simulink model "inanout"  (R2018a)
settings: Solver=FixedStepDiscrete  StartTime=0.0  StopTime=10.0  FixedStep=1e-4  RelTol=1e-3
InitFcn:
  | mbd_pnt_consistency_checks(bdroot(gcs));
undefined symbols (not defined in the file): B14, C10
libraries: mbd_pnt_ec_toolbox x6, simulink x2
settings Model: Creator=oolonthegreat  LastModifiedBy=oolonthegreat
settings DataIOCC: ExternalInput=off  InitialState=off  SaveOutput=off  SignalLogging=off  SaveTime=off
settings OptimizationCC: DefaultParameterBehavior=Inlined  EnhancedBackFolding=on  PassReuseOutputArgsAs=Individual arguments  OptimizeBlockOrder=speed  DifferentSizesBufferReuse=on  OptimizationCustomize=off
settings DebuggingCC: InheritedTsInSrcMsg=none  SingleTaskRateTransMsg=error  ParameterTunabilityLossMsg=error  UnconnectedInputMsg=error  UnconnectedOutputMsg=error  UnconnectedLineMsg=error  UnknownTsInhSupMsg=error
settings HardwareCC: ProdBitPerPointer=32  ProdBitPerSizeT=32  ProdBitPerPtrDiffT=32  ProdLargestAtomicInteger=Long  ProdLargestAtomicFloat=Double  ProdEndianess=BigEndian  ProdWordSize=32  ProdHWDeviceType=Motorola PowerPC
settings SFSimCC: MATLABDynamicMemAlloc=off
settings RTWCC: SystemTargetFile=mbd_pnt.tlc  MakeCommand=mbd_pnt_make_rtw COPY_MDLREF_INCLUDES=0  TemplateMakefile=mbd_pnt.tmf  PostCodeGenCommand=mbd_pnt_analyzegencode(buildInfo)  Description=Model Based Design Toolbox MPC574xP Code Generation Target  GenerateReport=on  IncludeHyperlinkInReport=on  LaunchReport=on  GenerateTraceInfo=on  GenerateTraceReport=on  GenerateTraceReportSl=on  GenerateTraceReportSf=on  GenerateTraceReportEml=on
settings CodeAppCC: ForceParamTrailComments=on  IgnoreCustomStorageClasses=off  OperatorAnnotations=on  SimulinkDataObjDesc=on  SFDataObjDesc=on  InsertBlockDesc=on
settings STFCustomTargetCC: TargetLangStandard=C99 (ISO)  MultiwordLength=256  CombineOutputUpdateFcns=on  SuppressErrorStatus=on  ERTCustomFileBanners=on  SupportContinuousTime=off  SupportNonInlinedSFcns=off  RemoveResetFunc=on  MATLABClassNameForMDSCustomization=Simulink.SoftwareTarget.ERTCustomization  GRTInterface=off  SystemTargetFile=mbd_pnt.tlc
settings ERTTargetCC: TargetLangStandard=C99 (ISO)  ParMdlRefBuildCompliant=off  CompOptLevelCompliant=off  ConcurrentExecutionCompliant=off  SuppressErrorStatus=on  ModelStepFunctionPrototypeControlCompliant=off  CPPClassGenCompliant=off  UseToolchainInfoCompliant=off  InlinedParameterPlacement=NonHierarchical  ERTCustomFileTemplate=example_file_process.tlc

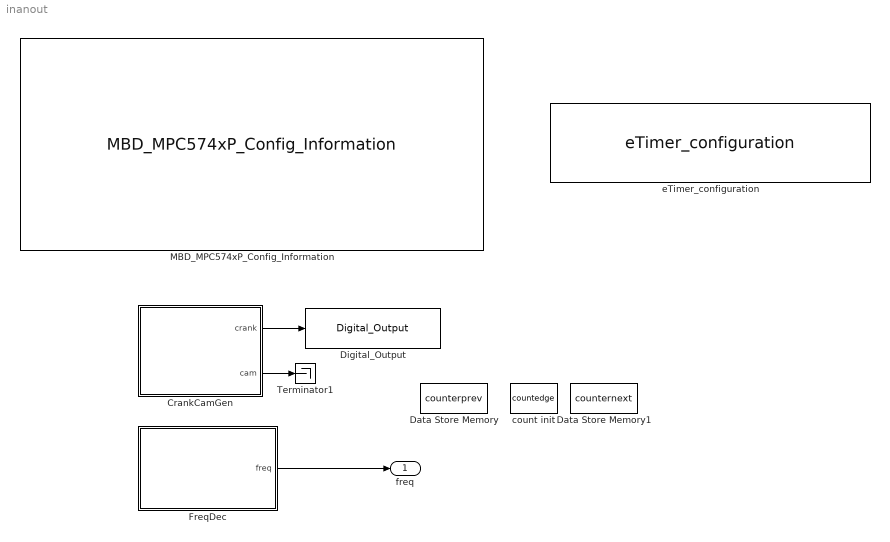
== system inanout ==
  CrankCamGen : Subsystem
  Data Store Memory : DataStoreMemory  DataStoreName=counterprev  ReadBeforeWriteMsg=warning  WriteAfterWriteMsg=warning  WriteAfterReadMsg=warning  ShowAdditionalParam=off  OutDataTypeStr=double
  Data Store Memory1 : DataStoreMemory  DataStoreName=counternext  ReadBeforeWriteMsg=warning  WriteAfterWriteMsg=warning  WriteAfterReadMsg=warning  ShowAdditionalParam=off  OutDataTypeStr=double
  Digital_Output : mbd_pnt_ec_toolbox/MPC574xP/Peripheral Interface Blocks/Digital_Output  gpio_outputs="42   : C10 :  [111] : [136] : [B14]"  pinNum=[111]  pcrNum=42
      settings: SourceProductName=Model Based Design Toolbox for MPC574xP
  FreqDec : Subsystem
  MBD_MPC574xP_Config_Information : mbd_pnt_ec_toolbox/MPC574xP/MBD_MPC574xP_Config_Information  disp_str=|  config_params=[]
      | System Clock : 200 MHz
      | Target : MPC5744P
      | Package : 144LQFP
      | XTAL Freq : 40 MHz
      | Compiler : S32 Design Studio
      | Target Type : FLASH
      | Global Interrupt Priority : 8
      | System Tick Interrupt Priority : 12
      | Freemaster : Serial1 (115200 Kbits)
      | Download Code after build : (COM5,115200)
      settings: SourceProductName=Model Based Design Toolbox for MPC574xP
  Terminator1 : Terminator
  count init : DataStoreMemory  DataStoreName=countedge  ReadBeforeWriteMsg=warning  WriteAfterWriteMsg=warning  WriteAfterReadMsg=warning  ShowAdditionalParam=off  OutDataTypeStr=double
  eTimer_configuration : mbd_pnt_ec_toolbox/MPC574xP/Motor Control Blocks/eTimer_configuration  SubModule=0  TimerChan=0  subMod=0  channel=0  CountMode=001 - Count rising edges of primary source  CNTMODE=1  CountOnce=0 - Count repeatedly  ONCE=0  CountLength=0 - Continue counting to roll over  LENGTH=0  CountDirection=0 - Count up  DIR=0  OutputEnable=0 - The external pin is configured as an input  OEN=0  CoChanInit=00 - Other channels cannot force re-initialization of this channel  COINIT=0  StopAction=0 - Output enable is unaffected by stop mode  STPEN=0  ReloadOnCapt=01 - Reload the counter on a capture 1 event  ROC=1  PrimarySource=11111 - IP Bus clock divide by 128 prescaler  PRISRC=31  PrimSrcPol=0 - True polarity  PIPS=0  SecondarySource=00000 - Counter #0 input pin  SECSRC=0  SecSrcPol=0 - True polarity  SIPS=0  FILT_CNT=0  FILT_PER=0  FILT=0  OutputMode=0000 - Software controlled  OUTMODE=0  OutputPol=0 - True polarity  OPS=0  MasterMode=0 - Disable broadcast of this channel output  MSTR=0  ForcedOutVal=0  VAL=0  CoForce=0 - Other channels cannot force this channel output  COFRC=0  CompLoad1=000 - COMP1 is never preload  CLC1=0  CompLoad2=000 - COMP2 is never preload  CLC2=0  CompareMode="00 - COMP1 and COMP2  are used when the counter is counting up"  CMPMODE=0  CaptMode1=10 - Capture rising edges  CPT1MODE=2  CaptMode2=00 - Capture disabled  CPT2MODE=0  OneShCaptMode=0 - Free running mode is selected  ONESHOT=0  CaptFIFO=0  CFWM=0  CNTRinit=0  COMP1init=0  COMP2init=0  mod0ch0pin="0     : A0   :  [73]   : [86]   : [P12]  input/output"  mod0ch1pin=None  mod0ch2pin=None  mod0ch3pin=None  mod0ch4pin=None  mod0ch5pin=None  mod1ch0pin=None  mod1ch1pin=None  mod1ch2pin=None  mod1ch3pin=None  mod1ch4pin=None  mod1ch5pin=None  mod2ch0pin=None  mod2ch1pin=None  mod2ch2pin=None  mod2ch3pin=None  mod2ch4pin=None  mod2ch5pin=None  pcrNum0=0  pcrNum1=255  pcrNum2=255  pcrNum3=255  pcrNum4=255  pcrNum5=255  TCFIE=off  TCF1IE=off  TCF2IE=off  TOFIE=off  IELFIE=off  IEHFIE=off  ICF1IE=on  ICF2IE=off  INTDMA=64
      settings: SourceProductName=Model Based Design Toolbox for MPC574xP
  freq : Outport
  wires:
  CrankCamGen/2(cam) -> Terminator1/1
  CrankCamGen/1(crank) -> Digital_Output/1
  FreqDec/1(freq) -> freq/1

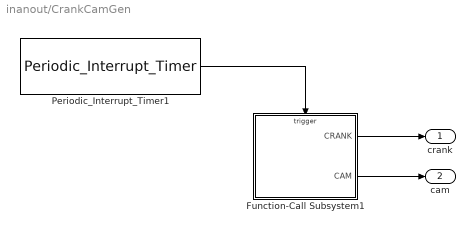
== system inanout/CrankCamGen ==
  Function-Call Subsystem1 : Subsystem  TreatAsAtomicUnit=on
  Periodic_Interrupt_Timer1 : mbd_pnt_ec_toolbox/MPC574xP/Utility Blocks/Periodic_Interrupt_Timer  pit_chan=1  pit_timeout=0.5  int_priority=15  pit_timeout_val=24999
      settings: SourceProductName=Model Based Design Toolbox for MPC574xP
  crank : Outport
  cam : Outport  Port=2
  wires:
  Periodic_Interrupt_Timer1/1 -> Function-Call Subsystem1/Trigger
  Function-Call Subsystem1/1(CRANK) -> crank/1
  Function-Call Subsystem1/2(CAM) -> cam/1

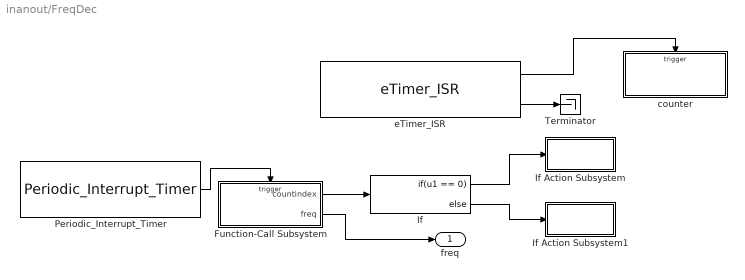
== system inanout/FreqDec ==
  Function-Call Subsystem : Subsystem  TreatAsAtomicUnit=on
  If : If  IfExpression=u1 == 0
  If Action Subsystem : Subsystem  TreatAsAtomicUnit=on
  If Action Subsystem1 : Subsystem  TreatAsAtomicUnit=on
  Periodic_Interrupt_Timer : mbd_pnt_ec_toolbox/MPC574xP/Utility Blocks/Periodic_Interrupt_Timer  pit_chan=1  pit_timeout=1000  int_priority=15  pit_timeout_val=49999999
      settings: SourceProductName=Model Based Design Toolbox for MPC574xP
  Terminator : Terminator
  counter : Subsystem  TreatAsAtomicUnit=on
  eTimer_ISR : mbd_pnt_ec_toolbox/MPC574xP/Motor Control Blocks/eTimer_ISR  SubModule=0  Timerchan=0  subMod=0  channel=0  isrPriority=14  isrPrio=14
      settings: SourceProductName=Model Based Design Toolbox for MPC574xP
  freq : Outport
  wires:
  eTimer_ISR/1 -> counter/Trigger
  Periodic_Interrupt_Timer/1 -> Function-Call Subsystem/Trigger
  Function-Call Subsystem/2(freq) -> freq/1
  Function-Call Subsystem/1(countindex) -> If/1
  If/1 -> If Action Subsystem/Action
  eTimer_ISR/2 -> Terminator/1
  If/2 -> If Action Subsystem1/Action

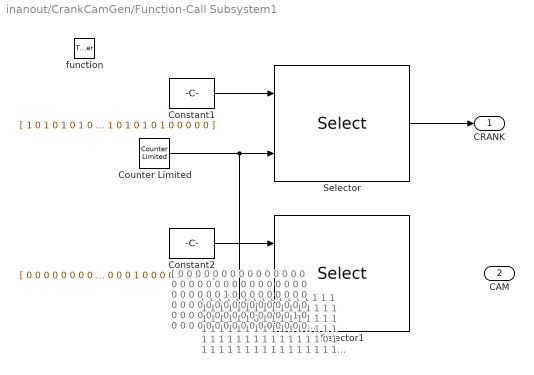
== system inanout/CrankCamGen/Function-Call Subsystem1 ==
  note: [ 1 1 1 1 1 1 1 1 1 1 1 1 1 1 1 1 1 1 1 1 1 1 1 1 1 1 1 1 1 1 1 1 1 1 1 1 1 0 1 1 1 1 1 1 1 1 1 1 1 1 1 1 1 1 1 1 1 1 1 1 1 1 1 1 1 1 1 1 1 1 1 1 1 1 1 1 1 0 1 1 1 1 1 1 1 1 1 1 1 1 1 1 1 1 1 1 1 1 1 1 1 1 1 1 1 1 1 1 1 1 1 1 1 1 1 1 1 0 1 1 1 1 1 1 1 1 1 1 1 1 1 1 1 1 1 1 1 1 1 1 1 1 1 1 1 1 1 1 1 1 1 1 1 1 1 1 1 0 1 1 1 1 1 1 1 1 1 1 1 1 1 1 1 1 1 1 1 1 1 1 1 1 1 1 1 1 1 1 1 1 1 1 1 1 1 1 1 0 1 1 1 1 1 1 1 1 1 1 1 1 1 1 1 1 1 1 1 1 1 1 1 1 1 1 1 1 1 1 1 1 1 0 1 1 1 1 1 0 1 1 ]
  note: [ 0 0 0 0 0 0 0 0 0 0 0 0 0 0 0 0 0 0 0 0 0 0 0 0 0 0 0 0 0 0 0 0 0 0 0 0 0 1 0 0 0 0 0 0 0 0 0 0 0 0 0 0 0 0 0 0 0 0 0 0 0 0 0 0 0 0 0 0 0 0 0 0 0 0 0 0 0 1 0 0 0 0 0 0 0 0 0 0 0 0 0 0 0 0 0 0 0 0 0 0 0 0 0 0 0 0 0 0 0 0 0 0 0 0 0 0 0 1 0 0 0 0 0 0 0 0 0 0 0 0 0 0 0 0 0 0 0 0 0 0 0 0 0 0 0 0 0 0 0 0 0 0 0 0 0 0 0 1 0 0 0 0 0 0 0 0 0 0 0 0 0 0 0 0 0 0 0 0 0 0 0 0 0 0 0 0 0 0 0 0 0 0 0 0 0 0 0 1 0 0 0 0 0 0 0 0 0 0 0 0 0 0 0 0 0 0 0 0 0 0 0 0 0 0 0 0 0 0 0 0 0 1 0 0 0 0 0 1 0 0 ]
  function : TriggerPort  TriggerType=function-call  VariantControl=Variant
  Constant1 : Constant  Value=[ 1 0 1 0 1 0 1 0 1 0 1 0 1 0 1 0 1 0 1 0 1 0 1 0 1 0 1 0 1 0 1 0 1 0 1 0 0 0 0 0 1 0 1 0 1 0 1 0 1 0 1 0 1 0 1 0 1 0 1 0 1 0 1 0 1 0 1 0 1 0 1 0 1 0 1 0 0 0 0 0 1 0 1 0 1 0 1 0 1 0 1 0 1 0 1 0 1 0 1 0 1 0 1 0 1 0 1 0 1 0 1 0 1 0 1 0 0 0 0 0 1 0 1 0 1 0 1 0 1 0 1 0 1 0 1 0 1 0 1 0 1 0 1 0 1 0 1 0 1 0 1 0 1 0 1 0 0 0 0 0 1 0 1 0 1 0 1 0 1 0 1 0 1 0 1 0 1 0 1 0 1 0 1 0 1 0 1 0 1 0 1 0 1 0 1 0 0 0 0 0 1 0 1 0 1 0 1 0 1 0 1 0 1 0 1 0 1 0 1 0 1 0 1 0 1 0 1 0 1 0 1 0 1 0 1 0 0 0 0 0 ]  OutDataTypeStr=boolean
  Constant2 : Constant  Value=[ 0 0 0 0 0 0 0 0 0 0 0 0 0 0 0 0 0 0 0 0 0 0 0 0 0 0 0 0 0 0 0 0 0 0 0 0 0 1 0 0 0 0 0 0 0 0 0 0 0 0 0 0 0 0 0 0 0 0 0 0 0 0 0 0 0 0 0 0 0 0 0 0 0 0 0 0 0 1 0 0 0 0 0 0 0 0 0 0 0 0 0 0 0 0 0 0 0 0 0 0 0 0 0 0 0 0 0 0 0 0 0 0 0 0 0 0 0 1 0 0 0 0 0 0 0 0 0 0 0 0 0 0 0 0 0 0 0 0 0 0 0 0 0 0 0 0 0 0 0 0 0 0 0 0 0 0 0 1 0 0 0 0 0 0 0 0 0 0 0 0 0 0 0 0 0 0 0 0 0 0 0 0 0 0 0 0 0 0 0 0 0 0 0 0 0 0 0 1 0 0 0 0 0 0 0 0 0 0 0 0 0 0 0 0 0 0 0 0 0 0 0 0 0 0 0 0 0 0 0 0 0 1 0 0 0 0 0 1 0 0 ]  OutDataTypeStr=boolean
  Counter Limited : simulink/Sources/Counter Limited  uplimit=239  tsamp=-1
  Selector : Selector  IndexMode=Zero-based  InputPortWidth=240  IndexOptions=Index vector (port)  Indices=[1 3]  OutputSizes=1
  Selector1 : Selector  IndexMode=Zero-based  InputPortWidth=240  IndexOptions=Index vector (port)  Indices=[1 3]  OutputSizes=1
  CRANK : Outport
  CAM : Outport  Port=2
  wires:
  Constant1/1 -> Selector/1
  Counter Limited/1 -> Selector1/2, Selector/2
  Constant2/1 -> Selector1/1
  Selector/1 -> CRANK/1

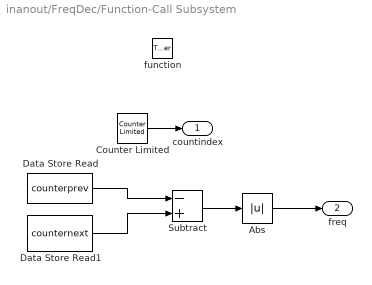
== system inanout/FreqDec/Function-Call Subsystem ==
  function : TriggerPort  TriggerType=function-call  VariantControl=Variant
  Abs : Abs
  Counter Limited : simulink/Sources/Counter Limited  uplimit=1  tsamp=-1
  Data Store Read : DataStoreRead  DataStoreName=counterprev
  Data Store Read1 : DataStoreRead  DataStoreName=counternext
  Subtract : Sum  Inputs=-+
  countindex : Outport
  freq : Outport  Port=2
  wires:
  Counter Limited/1 -> countindex/1
  Data Store Read/1 -> Subtract/1
  Data Store Read1/1 -> Subtract/2
  Subtract/1 -> Abs/1
  Abs/1 -> freq/1

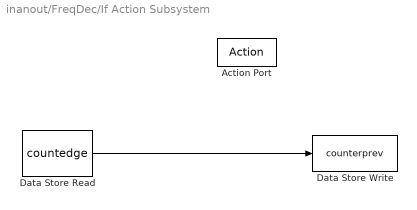
== system inanout/FreqDec/If Action Subsystem ==
  Action Port : ActionPort  ActionType=then
  Data Store Read : DataStoreRead  DataStoreName=countedge
  Data Store Write : DataStoreWrite  DataStoreName=counterprev
  wires:
  Data Store Read/1 -> Data Store Write/1

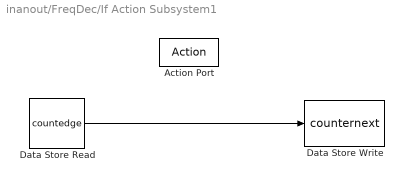
== system inanout/FreqDec/If Action Subsystem1 ==
  Action Port : ActionPort  ActionType=else
  Data Store Read : DataStoreRead  DataStoreName=countedge
  Data Store Write : DataStoreWrite  DataStoreName=counternext
  wires:
  Data Store Read/1 -> Data Store Write/1

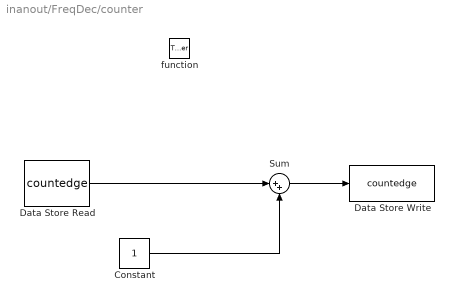
== system inanout/FreqDec/counter ==
  function : TriggerPort  TriggerType=function-call  VariantControl=Variant
  Constant : Constant  OutDataTypeStr=double
  Data Store Read : DataStoreRead  DataStoreName=countedge
  Data Store Write : DataStoreWrite  DataStoreName=countedge
  Sum : Sum  Inputs=|++
  wires:
  Constant/1 -> Sum/2
  Data Store Read/1 -> Sum/1
  Sum/1 -> Data Store Write/1
